simulink model "cartpole_pid_simulink"  (R2025a)
settings: Solver=ode45  StartTime=0.0  StopTime=10  MaxStep=0.001  RelTol=1e-3
values from neighbouring files (symbols this model uses):
  Fmax = 50    [auto_tune_pid.m]    (also in setup_lqr.m; setup_pd.m; setup_pid.m)
  Kd = 15    [setup_pd.m]    (also in setup_pid.m = 5)
  Ki = 0.5    [setup_pid.m]
  Kp = 80    [setup_pd.m]    (also in setup_pid.m = 120)
  Kv = -0.02    [setup_pid.m]
  Kx = -0.002    [setup_pid.m]
settings Model: Creator=Lee  LastModifiedBy=Lee

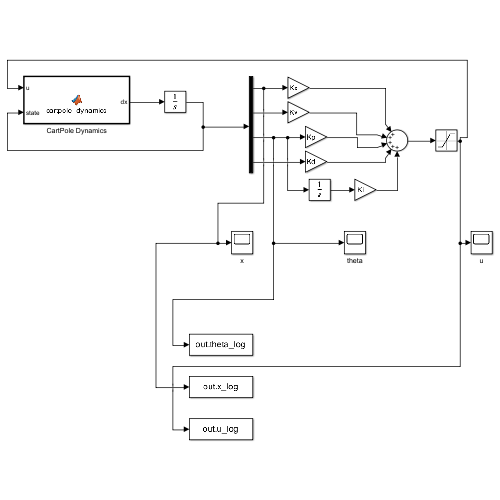
[thumbnail: Simulink's stored preview of the top-level diagram]
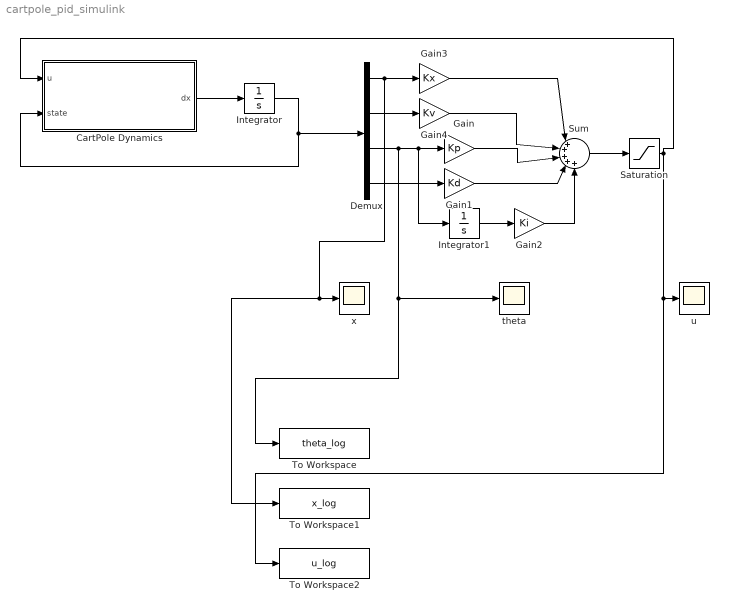
== system cartpole_pid_simulink ==
  CartPole Dynamics : MATLAB Function  TreatAsAtomicUnit=on
  Demux : Demux
  Gain : Gain  Gain=Kp
  Gain1 : Gain  Gain=Kd
  Gain2 : Gain  Gain=Ki
  Gain3 : Gain  Gain=Kx
  Gain4 : Gain  Gain=Kv
  Integrator : Integrator  InitialCondition=[0; 0; deg2rad(5); 0]
  Integrator1 : Integrator
  Saturation : Saturate  UpperLimit=Fmax  LowerLimit=-Fmax
  Sum : Sum  Inputs=|+++++
  To Workspace : ToWorkspace  VariableName=theta_log  SaveFormat=Timeseries  SampleTime=-1
  To Workspace1 : ToWorkspace  VariableName=x_log  SaveFormat=Timeseries  SampleTime=-1
  To Workspace2 : ToWorkspace  VariableName=u_log  SaveFormat=Timeseries  SampleTime=-1
  theta : Scope
      settings: ActiveDisplayYMinimum=-0.042562627672962386  ActiveDisplayYMaximum=0.10169191707445857
  u : Scope
      settings: ActiveDisplayYMinimum=-5.9875339390051678  ActiveDisplayYMaximum=12.300809895407216  DataLoggingVariableName=ScopeData2
  x : Scope
      settings: ActiveDisplayYMinimum=-0.056017995257456571  ActiveDisplayYMaximum=0.50416195731710922
  wires:
  CartPole Dynamics/1(dx) -> Integrator/1
  Integrator/1 -> Demux/1, CartPole Dynamics/2(state)
  Demux/3 -> Integrator1/1, Gain/1, To Workspace/1, theta/1
  Demux/4 -> Gain1/1
  Sum/1 -> Saturation/1
  Saturation/1 -> To Workspace2/1, u/1, CartPole Dynamics/1(u)
  Demux/1 -> Gain3/1, To Workspace1/1, x/1
  Integrator1/1 -> Gain2/1
  Demux/2 -> Gain4/1
  Gain3/1 -> Sum/1
  Gain4/1 -> Sum/2
  Gain/1 -> Sum/3
  Gain1/1 -> Sum/4
  Gain2/1 -> Sum/5

== matlab function cartpole_pid_simulink/CartPole Dynamics ==
  data: u input; dx output; state input
function dx = cartpole_dynamics(u, state)

M = 1.0;
m = 0.1;
l = 0.5;
g = 9.8;

x = state(1);
x_dot = state(2);
theta = state(3);
theta_dot = state(4);

den = M + m*sin(theta)^2;

x_ddot = (u + m * sin(theta) * (l * theta_dot^2 - g * cos(theta))) / den;

theta_ddot = (-u * cos(theta) - m * l * theta_dot^2 * sin(theta) * cos(theta) + (M + m) * g * sin(theta)) / (l * den);

dx = zeros(4,1);
dx(1) = x_dot;
dx(2) = x_ddot;
dx(3) = theta_dot;
dx(4) = theta_ddot;

end
